simulink model "TemplateNoLineal2_2015b"  (R2021a)
settings: Solver=ode4  StartTime=0.0  StopTime=10.0  FixedStep=0.0001  RelTol=1e-3
libraries: cstblocks x1
settings Model: Creator=aghersin  LastModifiedBy=Euge Etcheverry
settings SolverCC: AlgebraicLoopSolver=TrustRegion
settings DataIOCC: ReturnWorkspaceOutputs=off
settings OptimizationCC: LifeSpan=inf
settings DebuggingCC: SFExecutionAtInitializationDiag=none  SFMachineParentedDataDiag=warning  ArithmeticOperatorsInVariantConditions=warning
settings SFSimCC: SimUseLocalCustomCode=off  CustomCodeUndefinedFunction=UseInterfaceOnly
settings RTWCC: RTWUseLocalCustomCode=off
settings CodeAppCC: StateflowObjectComments=on

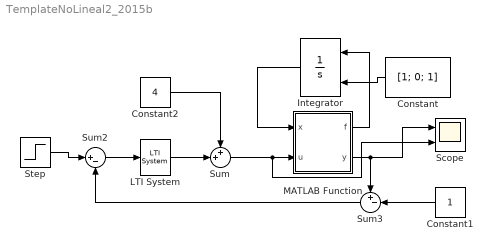
== system TemplateNoLineal2_2015b ==
  Constant : Constant  Value=[1; 0; 1]
  Constant1 : Constant
  Constant2 : Constant  Value=4
  Integrator : Integrator  InitialConditionSource=external
  LTI System : cstblocks/LTI System  sys=Cd  IC=[]
  MATLAB Function : MATLAB Function  TreatAsAtomicUnit=on
  Scope : Scope  NumInputPorts=2
  Step : Step  After=0.5  SampleTime=0
  Sum : Sum  Inputs=++|
  Sum2 : Sum  Inputs=|+-
  Sum3 : Sum  Inputs=+-|
  wires:
  Integrator/1 -> MATLAB Function/1(x)
  MATLAB Function/1(f) -> Integrator/1
  Constant/1 -> Integrator/2
  MATLAB Function/2(y) -> Sum3/1, Scope/1
  Constant1/1 -> Sum3/2
  Constant2/1 -> Sum/1
  Sum2/1 -> LTI System/1
  Sum3/1 -> Sum2/2
  LTI System/1 -> Sum/2
  Sum/1 -> Scope/2, MATLAB Function/2(u)
  Step/1 -> Sum2/1

== matlab function TemplateNoLineal2_2015b/MATLAB Function ==
  data: x input; u input; f output; y output
function [f,y] = fcn(x,u)
g = 10;
m = 0.1;
L = 1e-2;
R = 4;

f1=x(2);
f2=g-x(3)/(m*x(1));
f3=u/L-x(3)*R/L;

f=[f1;f2;f3];

y=x(1);
